simulink model "VINS"  (R2018a)
settings: Solver=FixedStepDiscrete  StartTime=0.0  StopTime=inf  FixedStep=1/Fs  RelTol=1e-3  EnableMultiTasking=on
PreLoadFcn:
  | modelDef = getModelDef(calibrateSFMA);
  | 
  | %imuPar = getImuPar('lmvpUncalibrated');
  | 
  | timeMatchThreshold = 1000;
undefined symbols (not defined in the file or in its folder): beep, dejitter_on, Fs, homogeneous3x4Transform_k_kmin1, imuLocationMm, imuPar, numStates, simData, tstamp_k_us, tstamp_kmin1_us
libraries: simulink x69, dspmtrx3 x35, dspindex x9, vrlib x7, dspstat3 x7, dspinverses x6, dspsigops x5, dspmathops x2, rtwdemowidgets x1, dspfactors x1, simulink_extras x1
(part 5 of 6)

== system VINS/measUpdate/absolutePoseUpdate/applyErrors/applyXstateErrors/reOrthonormalization ==
  note: from http://www.dtic.mil/dtic/tr/fulltext/u2/p003621.pdf page 12
  note: Cfixed = C + 0.5(I-CC')C
  In1 : Inport
  C*C' : Product  Multiplication=Matrix(*)
  C*C'1 : Product  Multiplication=Matrix(*)
  Constant : Constant  Value=eye(3)  OutDataTypeStr=Inherit: Inherit via back propagation
  Gain : Gain  Gain=1/2
  Permute Dimensions : PermuteDimensions
  Sum : Sum  Inputs=|++
  Sum1 : Sum  Inputs=|+-
  Out1 : Outport
  wires:
  In1/1 -> Permute Dimensions/1, C*C'/1, C*C'1/2, Sum/1
  Sum/1 -> Out1/1
  Permute Dimensions/1 -> C*C'/2
  C*C'/1 -> Sum1/2
  Constant/1 -> Sum1/1
  Gain/1 -> Sum/2
  Sum1/1 -> C*C'1/1
  C*C'1/1 -> Gain/1

== system VINS/measUpdate/absolutePoseUpdate/applyErrors/applyXstateErrors/updateAccelBiases ==
  In1 : Inport
  Enable : EnablePort
  Data Store Read5 : DataStoreRead  DataStoreName=df
  Data Store Write5 : DataStoreWrite  DataStoreName=df
  Sum4 : Sum  Inputs=++|
  wires:
  In1/1 -> Sum4/1
  Data Store Read5/1 -> Sum4/2
  Sum4/1 -> Data Store Write5/1

== system VINS/measUpdate/absolutePoseUpdate/applyErrors/applyXstateErrors/updateAccelSfma ==
  In1 : Inport
  Enable : EnablePort
  " LU Inverse" : dspinverses/ LU Inverse
      settings: SourceProductName=DSP System Toolbox
  Bias : Bias  Bias=eye(3)
  Data Store Read6 : DataStoreRead  DataStoreName=Macc
  Data Store Write6 : DataStoreWrite  DataStoreName=Macc
  Data Store Write9 : DataStoreWrite  DataStoreName=IplusMinv_acc
  Reshape : Reshape  OutputDimensionality=Customize  OutputDimensions=[3,3]
  Sum5 : Sum  Inputs=++|
  wires:
  " LU Inverse"/1 -> Data Store Write9/1
  Bias/1 -> " LU Inverse"/1
  In1/1 -> Reshape/1
  Reshape/1 -> Sum5/1
  Data Store Read6/1 -> Sum5/2
  Sum5/1 -> Data Store Write6/1, Bias/1

== system VINS/measUpdate/absolutePoseUpdate/applyErrors/applyXstateErrors/updateGyroGsensitivity ==
  In1 : Inport
  Enable : EnablePort
  Data Store Read7 : DataStoreRead  DataStoreName=Ggyr
  Data Store Write7 : DataStoreWrite  DataStoreName=Ggyr
  Reshape1 : Reshape  OutputDimensionality=Customize  OutputDimensions=[3,3]
  Sum6 : Sum  Inputs=++|
  wires:
  Data Store Read7/1 -> Sum6/2
  Reshape1/1 -> Sum6/1
  In1/1 -> Reshape1/1
  Sum6/1 -> Data Store Write7/1

== system VINS/measUpdate/absolutePoseUpdate/applyErrors/applyXstateErrors/updateGyroSfma ==
  In1 : Inport
  Enable : EnablePort
  " LU Inverse1" : dspinverses/ LU Inverse
      settings: SourceProductName=DSP System Toolbox
  Bias1 : Bias  Bias=eye(3)
  Data Store Read7 : DataStoreRead  DataStoreName=Mgyr
  Data Store Write7 : DataStoreWrite  DataStoreName=Mgyr
  Data Store Write8 : DataStoreWrite  DataStoreName=IplusMinv_gyr
  Reshape1 : Reshape  OutputDimensionality=Customize  OutputDimensions=[3,3]
  Sum6 : Sum  Inputs=++|
  wires:
  " LU Inverse1"/1 -> Data Store Write8/1
  Bias1/1 -> " LU Inverse1"/1
  Data Store Read7/1 -> Sum6/2
  Reshape1/1 -> Sum6/1
  In1/1 -> Reshape1/1
  Sum6/1 -> Data Store Write7/1, Bias1/1

== system VINS/measUpdate/relativePoseUpdate/applyErrors/applyErrors/For Each Subsystem ==
  delayedPoseCorrections : Inport  Partition=on  PartitionDimension=1  PartitionWidth=6  PartitionOffset=0
  C_c_n_list_in : Inport  Port=2  Partition=on  PartitionDimension=3  PartitionWidth=1  PartitionOffset=0
  r_c_n_list_in : Inport  Port=3  Partition=on  PartitionDimension=3  PartitionWidth=1  PartitionOffset=0
  Demux : Demux  Outputs=[3 3]
  For Each : ForEach  DisableCoverage=on  IndexMode=One-based
  Product2 : Product  Multiplication=Matrix(*)
  Sum : Sum  Inputs=++|
  Sum2 : Sum  Inputs=-+|
  reOrthonormalization : Subsystem  TreatAsAtomicUnit=on
  skew : MATLAB Function  TreatAsAtomicUnit=on
  C_c_n_list : Outport  ConcatenationDimension=3
  r_c_n_list : Outport  Port=2  ConcatenationDimension=3
  wires:
  delayedPoseCorrections/1 -> Demux/1
  Product2/1 -> Sum/1
  C_c_n_list_in/1 -> Sum/2, Product2/2
  reOrthonormalization/1(Out1) -> C_c_n_list/1
  skew/1(res) -> Product2/1  "[phi X]"
  Sum2/1 -> r_c_n_list/1
  r_c_n_list_in/1 -> Sum2/2
  Demux/1 -> skew/1(inp_vr)  "phi rotation errors"
  Demux/2 -> Sum2/1
  Sum/1 -> reOrthonormalization/1(In1)

== system VINS/measUpdate/relativePoseUpdate/applyErrors/applyErrors/applyXstateErrors ==
  errorStateEstimates : Inport
  Constant : Constant  Value=modelDef.trackGyroSfma
  Constant1 : Constant  Value=modelDef.trackAccelSfma
  Constant2 : Constant  Value=modelDef.trackAccelBiases
  Constant3 : Constant  Value=modelDef.trackGyroGsens
  Data Store Read1 : DataStoreRead  DataStoreName=dw
  Data Store Read2 : DataStoreRead  DataStoreName=Cbn
  Data Store Read3 : DataStoreRead  DataStoreName=rnav
  Data Store Read4 : DataStoreRead  DataStoreName=vnav
  Data Store Write1 : DataStoreWrite  DataStoreName=Cbn
  Data Store Write2 : DataStoreWrite  DataStoreName=dw
  Data Store Write3 : DataStoreWrite  DataStoreName=rnav
  Data Store Write4 : DataStoreWrite  DataStoreName=vnav
  Multiport Selector : dspindex/Multiport Selector  rowsOrCols=Rows  idxCellArray={ 1:3, 4:6, 7:9, 10:12, 13:15, 16:24, 25:33, 34:42 }  idxErrMode=Clip Index
  Product2 : Product  Multiplication=Matrix(*)
  Scope{,1..3} (4 alike) : Scope
  Sum : Sum  Inputs=++|
  Sum1 : Sum  Inputs=++|
  Sum2 : Sum  Inputs=-+|
  Sum3 : Sum  Inputs=-+|
  reOrthonormalization : Subsystem  TreatAsAtomicUnit=on
  skew : MATLAB Function  TreatAsAtomicUnit=on
  updateAccelBiases : Subsystem
  updateAccelSfma : Subsystem
  updateGyroGsensitivity : Subsystem
  updateGyroSfma : Subsystem
  wires:
  Multiport Selector/4 -> Sum3/1, Scope2/1
  Multiport Selector/3 -> Sum2/1, Scope1/1
  Sum3/1 -> Data Store Write4/1
  Data Store Read4/1 -> Sum3/2
  Data Store Read3/1 -> Sum2/2
  Sum2/1 -> Data Store Write3/1
  errorStateEstimates/1 -> Multiport Selector/1
  Multiport Selector/2 -> Sum1/1, Scope/1  "gyro bias errors"
  Sum1/1 -> Data Store Write2/1
  Data Store Read1/1 -> Sum1/2
  Multiport Selector/1 -> skew/1(inp_vr)  "phi rotation errors"
  reOrthonormalization/1(Out1) -> Data Store Write1/1
  Data Store Read2/1 -> Sum/2, Product2/2
  Sum/1 -> reOrthonormalization/1(In1)
  Product2/1 -> Sum/1
  skew/1(res) -> Product2/1  "[phi X]"
  Constant/1 -> updateGyroSfma/Enable
  Multiport Selector/6 -> updateGyroSfma/1(In1)
  Constant1/1 -> updateAccelSfma/Enable
  Multiport Selector/7 -> updateAccelSfma/1(In1)
  Multiport Selector/5 -> updateAccelBiases/1(In1), Scope3/1
  Constant2/1 -> updateAccelBiases/Enable
  Constant3/1 -> updateGyroGsensitivity/Enable
  Multiport Selector/8 -> updateGyroGsensitivity/1(In1)

== system VINS/measUpdate/relativePoseUpdate/get row indices/validateRecency/previousIndex ==
  idx2 : Inport
  Constant : Constant  Value=modelDef.maxNumDelayedPoses
  Constant1 : Constant  Value=uint8(1)
  Sum : Sum  Inputs=|-+
  Switch : Switch  Threshold=uint8(2)
  idx1 : Outport
  wires:
  idx2/1 -> Sum/2, Switch/2
  Constant/1 -> Switch/3
  Constant1/1 -> Sum/1
  Sum/1 -> Switch/1
  Switch/1 -> idx1/1  "idx1"

== system VINS/measUpdate/relativePoseUpdate/get row indices/validateRecency/previousIndex1 ==
  idx2 : Inport
  Constant : Constant  Value=modelDef.maxNumDelayedPoses
  Constant1 : Constant  Value=uint8(1)
  Sum : Sum  Inputs=|-+
  Switch : Switch  Threshold=uint8(2)
  idx1 : Outport
  wires:
  Switch/1 -> idx1/1  "idx1"
  Sum/1 -> Switch/1
  Constant1/1 -> Sum/1
  Constant/1 -> Switch/3
  idx2/1 -> Switch/2, Sum/2

== system VINS/measUpdate/relativePoseUpdate/updateCovariance/repairCovarianceAndWrite/lowerBoundDiagonal and reconstruct ==
  note: lower bound sigmas:
      |
      | phi:  1e-4 rad
      | dw:  20 deg/hr =1e-4 rad/s
      | dr: 1e-4 m
      | dv: 1e-4 m/s
      | df: max(imuPar.accelAlignUncert, imuPar.accelScaleUncert) * 9.8 m/s/s
  LDL' : Inport
  Create Diagonal Matrix : dspmtrx3/Create Diagonal Matrix
      settings: SourceProductName=DSP System Toolbox  SourceProductBaseCode=DS
  Extract Diagonal : dspmtrx3/Extract Diagonal
      settings: SourceProductName=DSP System Toolbox  SourceProductBaseCode=DS
  Extract Triangular Matrix : dspmtrx3/Extract Triangular Matrix  fcn=Lower  SimulateUsing=Code generation
      settings: SourceProductName=DSP System Toolbox  SourceProductBaseCode=DS
  Math Function : Math  Operator=square  SaturateOnIntegerOverflow=on
  Matrix Multiply : Product  Inputs=3  Multiplication=Matrix(*)
  Max : MinMax  Function=max  Inputs=2
  MinMax : MinMax
  MinMax1 : MinMax  Function=max
  Overwrite Values : dspmtrx3/Overwrite Values  OverWriteDiag=Diagonal  valFrom2ndIP=Second input port  ConstValue=0  RowSpan=Range of rows  RowStartMode=First  RowStartIndex=1  RowEndMode=Last  RowEndIndex=1  ColSpan=Range of columns  ColStartMode=First  ColStartIndex=1  ColEndMode=Last  ColEndIndex=1  DiagSpan=All elements  DiagStartMode=Index  DiagStartIndex=2  DiagEndMode=Index  DiagEndIndex=4
      settings: SourceProductName=DSP System Toolbox  SourceProductBaseCode=DS
  Permute Dimensions : PermuteDimensions
  Scope : Scope  NumInputPorts=2
  lowerBoundSigmas : Constant  Value="[1e-4 * ones(1,12)  9.8*max(imuPar.accelAlignUncert, imuPar.accelScaleUncert) * ones(1,3*modelDef.trackAccelBiases)   1e-4 * ones(1,modelDef.maxNumDelayedPoses*modelDef.statesPerDelayedPose)]"  OutDataTypeStr=Inherit: Inherit via back propagation
  ones size of diagonal : Product  Inputs=*/
  ones size of diagonal1 : Product  Inputs=*/
  rcond? : Scope
  P : Outport
  wires:
  Extract Diagonal/1 -> MinMax1/1, MinMax/1, Max/1, ones size of diagonal/2, ones size of diagonal/1
  Math Function/1 -> Max/2
  lowerBoundSigmas/1 -> Math Function/1
  LDL'/1 -> Extract Triangular Matrix/1, Extract Diagonal/1
  Extract Triangular Matrix/1 -> Overwrite Values/1
  ones size of diagonal/1 -> Overwrite Values/2
  Overwrite Values/1 -> Permute Dimensions/1, Matrix Multiply/1  "L"
  Matrix Multiply/1 -> P/1
  Permute Dimensions/1 -> Matrix Multiply/3  "L'"
  Create Diagonal Matrix/1 -> Matrix Multiply/2
  MinMax/1 -> ones size of diagonal1/1, Scope/1
  MinMax1/1 -> ones size of diagonal1/2, Scope/2
  ones size of diagonal1/1 -> rcond?/1
  Max/1 -> Create Diagonal Matrix/1

== system VINS/measUpdate/relativePoseUpdate/updateCovariance/writeCovariances/lowerBoundStates ==
  note: lower bound sigmas:
      |
      | phi:  1e-4 rad
      | dw:  20 deg/hr =1e-4 rad/s
      | dr: 1e-4 m
      | dv: 1e-4 m/s
      | df: max(imuPar.accelAlignUncert, imuPar.accelScaleUncert) * 9.8 m/s/s
  In1 : Inport
  Extract Diagonal : dspmtrx3/Extract Diagonal
      settings: SourceProductName=DSP System Toolbox  SourceProductBaseCode=DS
  Math Function : Math  Operator=square  SaturateOnIntegerOverflow=on
  Max : MinMax  Function=max  Inputs=2
  Overwrite Values : dspmtrx3/Overwrite Values  OverWriteDiag=Diagonal  valFrom2ndIP=Second input port  ConstValue=0  RowSpan=Range of rows  RowStartMode=First  RowStartIndex=1  RowEndMode=Last  RowEndIndex=1  ColSpan=Range of columns  ColStartMode=First  ColStartIndex=1  ColEndMode=Last  ColEndIndex=1  DiagSpan=All elements  DiagStartMode=Index  DiagStartIndex=2  DiagEndMode=Index  DiagEndIndex=4
      settings: SourceProductName=DSP System Toolbox  SourceProductBaseCode=DS
  lowerBoundSigmas : Constant  Value="[1e-4 * ones(1,12)  9.8*max(imuPar.accelAlignUncert, imuPar.accelScaleUncert) * ones(1,3)]"  OutDataTypeStr=Inherit: Inherit via back propagation
  Out1 : Outport
  wires:
  In1/1 -> Overwrite Values/1, Extract Diagonal/1
  lowerBoundSigmas/1 -> Math Function/1
  Extract Diagonal/1 -> Max/1
  Math Function/1 -> Max/2
  Max/1 -> Overwrite Values/2
  Overwrite Values/1 -> Out1/1

== system VINS/measUpdate/relativePoseUpdate/updateCovariance/writeCovariances/lowerBoundStates1 ==
  note: lower bound sigmas:
      |
      | phi:  1e-4 rad
      | dw:  20 deg/hr =1e-4 rad/s
      | dr: 1e-4 m
      | dv: 1e-4 m/s
      | df: max(imuPar.accelAlignUncert, imuPar.accelScaleUncert) * 9.8 m/s/s
  In1 : Inport
  Extract Diagonal : dspmtrx3/Extract Diagonal
      settings: SourceProductName=DSP System Toolbox  SourceProductBaseCode=DS
  Math Function : Math  Operator=square  SaturateOnIntegerOverflow=on
  Max : MinMax  Function=max  Inputs=2
  Overwrite Values : dspmtrx3/Overwrite Values  OverWriteDiag=Diagonal  valFrom2ndIP=Second input port  ConstValue=0  RowSpan=Range of rows  RowStartMode=First  RowStartIndex=1  RowEndMode=Last  RowEndIndex=1  ColSpan=Range of columns  ColStartMode=First  ColStartIndex=1  ColEndMode=Last  ColEndIndex=1  DiagSpan=All elements  DiagStartMode=Index  DiagStartIndex=2  DiagEndMode=Index  DiagEndIndex=4
      settings: SourceProductName=DSP System Toolbox  SourceProductBaseCode=DS
  lowerBoundSigmas : Constant  Value="[  1e-4 * ones(1,modelDef.maxNumDelayedPoses*modelDef.statesPerDelayedPose) ]"  OutDataTypeStr=Inherit: Inherit via back propagation
  Out1 : Outport
  wires:
  Overwrite Values/1 -> Out1/1
  Max/1 -> Overwrite Values/2
  Math Function/1 -> Max/2
  Extract Diagonal/1 -> Max/1
  lowerBoundSigmas/1 -> Math Function/1
  In1/1 -> Extract Diagonal/1, Overwrite Values/1

== system VINS/measUpdate/relocalize/Subsystem/setPosition/DT police3 ==
  In1 : Inport
  Data Store Read : DataStoreRead  DataStoreName=DataTypeRef
  Data Type Duplicate : DataTypeDuplicate
  wires:
  Data Store Read/1 -> Data Type Duplicate/1
  In1/1 -> Data Type Duplicate/2

== system VINS/measUpdate/relativePoseUpdate/applyErrors/applyErrors/For Each Subsystem/reOrthonormalization ==
  note: Cfixed = C + 0.5(I-CC')C
  note: from http://www.dtic.mil/dtic/tr/fulltext/u2/p003621.pdf page 12
  In1 : Inport
  C*C' : Product  Multiplication=Matrix(*)
  C*C'1 : Product  Multiplication=Matrix(*)
  Constant : Constant  Value=eye(3)  OutDataTypeStr=Inherit: Inherit via back propagation
  Gain : Gain  Gain=1/2
  Permute Dimensions : PermuteDimensions
  Sum : Sum  Inputs=|++
  Sum1 : Sum  Inputs=|+-
  Out1 : Outport
  wires:
  C*C'1/1 -> Gain/1
  Sum1/1 -> C*C'1/1
  Gain/1 -> Sum/2
  Constant/1 -> Sum1/1
  C*C'/1 -> Sum1/2
  Permute Dimensions/1 -> C*C'/2
  Sum/1 -> Out1/1
  In1/1 -> Sum/1, C*C'1/2, C*C'/1, Permute Dimensions/1

== system VINS/measUpdate/relativePoseUpdate/applyErrors/applyErrors/applyXstateErrors/reOrthonormalization ==
  note: Cfixed = C + 0.5(I-CC')C
  note: from http://www.dtic.mil/dtic/tr/fulltext/u2/p003621.pdf page 12
  In1 : Inport
  C*C' : Product  Multiplication=Matrix(*)
  C*C'1 : Product  Multiplication=Matrix(*)
  Constant : Constant  Value=eye(3)  OutDataTypeStr=Inherit: Inherit via back propagation
  Gain : Gain  Gain=1/2
  Permute Dimensions : PermuteDimensions
  Sum : Sum  Inputs=|++
  Sum1 : Sum  Inputs=|+-
  Out1 : Outport
  wires:
  C*C'1/1 -> Gain/1
  Sum1/1 -> C*C'1/1
  Gain/1 -> Sum/2
  Constant/1 -> Sum1/1
  C*C'/1 -> Sum1/2
  Permute Dimensions/1 -> C*C'/2
  Sum/1 -> Out1/1
  In1/1 -> Sum/1, C*C'1/2, C*C'/1, Permute Dimensions/1

== system VINS/measUpdate/relativePoseUpdate/applyErrors/applyErrors/applyXstateErrors/updateAccelBiases ==
  In1 : Inport
  Enable : EnablePort
  Data Store Read5 : DataStoreRead  DataStoreName=df
  Data Store Write5 : DataStoreWrite  DataStoreName=df
  Sum4 : Sum  Inputs=++|
  wires:
  Sum4/1 -> Data Store Write5/1
  Data Store Read5/1 -> Sum4/2
  In1/1 -> Sum4/1

== system VINS/measUpdate/relativePoseUpdate/applyErrors/applyErrors/applyXstateErrors/updateAccelSfma ==
  In1 : Inport
  Enable : EnablePort
  " LU Inverse" : dspinverses/ LU Inverse
      settings: SourceProductName=DSP System Toolbox
  Bias : Bias  Bias=eye(3)
  Data Store Read6 : DataStoreRead  DataStoreName=Macc
  Data Store Write6 : DataStoreWrite  DataStoreName=Macc
  Data Store Write9 : DataStoreWrite  DataStoreName=IplusMinv_acc
  Reshape : Reshape  OutputDimensionality=Customize  OutputDimensions=[3,3]
  Sum5 : Sum  Inputs=++|
  wires:
  Sum5/1 -> Bias/1, Data Store Write6/1
  Data Store Read6/1 -> Sum5/2
  Reshape/1 -> Sum5/1
  In1/1 -> Reshape/1
  Bias/1 -> " LU Inverse"/1
  " LU Inverse"/1 -> Data Store Write9/1

== system VINS/measUpdate/relativePoseUpdate/applyErrors/applyErrors/applyXstateErrors/updateGyroGsensitivity ==
  In1 : Inport
  Enable : EnablePort
  Data Store Read7 : DataStoreRead  DataStoreName=Ggyr
  Data Store Write7 : DataStoreWrite  DataStoreName=Ggyr
  Reshape1 : Reshape  OutputDimensionality=Customize  OutputDimensions=[3,3]
  Sum6 : Sum  Inputs=++|
  wires:
  Sum6/1 -> Data Store Write7/1
  In1/1 -> Reshape1/1
  Reshape1/1 -> Sum6/1
  Data Store Read7/1 -> Sum6/2

== system VINS/measUpdate/relativePoseUpdate/applyErrors/applyErrors/applyXstateErrors/updateGyroSfma ==
  In1 : Inport
  Enable : EnablePort
  " LU Inverse1" : dspinverses/ LU Inverse
      settings: SourceProductName=DSP System Toolbox
  Bias1 : Bias  Bias=eye(3)
  Data Store Read7 : DataStoreRead  DataStoreName=Mgyr
  Data Store Write7 : DataStoreWrite  DataStoreName=Mgyr
  Data Store Write8 : DataStoreWrite  DataStoreName=IplusMinv_gyr
  Reshape1 : Reshape  OutputDimensionality=Customize  OutputDimensions=[3,3]
  Sum6 : Sum  Inputs=++|
  wires:
  Sum6/1 -> Bias1/1, Data Store Write7/1
  In1/1 -> Reshape1/1
  Reshape1/1 -> Sum6/1
  Data Store Read7/1 -> Sum6/2
  Bias1/1 -> " LU Inverse1"/1
  " LU Inverse1"/1 -> Data Store Write8/1

== matlab function VINS/stilltimes/updateStilltimeTight ==
  data: w input; stilltime output; f input; Dt input; favgs output; wavgs output; wsigma input; fsigma input
function [stilltime, favgs, wavgs] = update_stilltime(w, f, Dt, wsigma, fsigma)

persistent stillt wavg favg stillcycles wsigmas fsigmas;

if isempty(wavg)
    stillt = cast(0, 'like', w);
    stillcycles = cast(0, 'like', w);
    wavg = w;
    favg = f;
    wsigmas = wsigma*cast([1;1;1], 'like', w);
    fsigmas = fsigma*cast([1;1;1], 'like', w);
end

if all(abs(f-favg) < 3*fsigmas) && all(abs(w-wavg) < 3*wsigmas)  % increment the stilltimes
    stillt = stillt + Dt;
    stillcycles = stillcycles + cast(1, 'like', w);
%     % simple recursive mean (weighting all the samples equally):
%     wavg = ((stillcycles-1)*wavg + w)/stillcycles;
%     favg = ((stillcycles-1)*favg + f)/stillcycles;

%     % recursive mean with each sample weighted by the stillcycles when it came in:
%     wavg = ((stillcycles-1)*wavg + 2*w)/(stillcycles+1);
%     favg = ((stillcycles-1)*favg + 2*f)/(stillcycles+1);

    % start with stillcycles weighting and switch back to simple recursive mean after 1 second to reduce noise:
    if stillt < 1
        wavg = ((stillcycles-cast(1, 'like', w))*wavg + 2*w)/(stillcycles+cast(1, 'like', w));
        favg = ((stillcycles-1)*favg + 2*f)/(stillcycles+1);
    else
        wavg = ((stillcycles-1)*wavg + w)/stillcycles;
        favg = ((stillcycles-1)*favg + f)/stillcycles;
    end        
else  %reset stilltime
    stillt = cast(0, 'like', w);
    stillcycles = cast(0, 'like', w);
    wavg = w;
    favg = f;
end    

stilltime = stillt;
favgs = favg;
wavgs = wavg;

== matlab function VINS/reportOutputs/MATLAB Function3 ==
  data: Cbn input; eul output size=[3,1]
function eul = dcm2euler(Cbn)

%DCM is Cbn (transforms vectors from b to n)
%eul defined as zyx sequence (yaw,pitch,roll),  but listed in
%roll,pitch,yaw order


pitch=asin(-Cbn(3,1));  %pitch is assumed to be [-pi pi]. singular at pi. use ad-hoc methods to remedy this deficiency
roll=atan2(Cbn(3,2), Cbn(3,3));
heading = atan2(Cbn(2,1), Cbn(1,1));
eul=[roll;pitch;heading];

== matlab function VINS/measUpdate/gravity meas update/update the Cbn and b_g with the errors/MATLAB Function ==
  data: inp_vr input; res output
function res=skew(inp_vr)
res=[0 			-inp_vr(3)	inp_vr(2); ...
     inp_vr(3)	0			-inp_vr(1);...
	 -inp_vr(2)	inp_vr(1)	0];

== matlab function VINS/measUpdate/gravity meas update/MATLAB Function1 ==
  data: S output; P input; K output; H input; R input
function [S,K] = calcKalmanGain(P, H, R)

PHT = P*H';
S = H*PHT + R;
K = PHT/S;

== matlab function VINS/uncomment and set zero noise for verification/plot errors/MATLAB Function3 ==
  data: Cbn input; eul output size=[3,1]
function eul = dcm2euler(Cbn)

%DCM is Cbn (transforms vectors from b to n)
%eul defined as zyx sequence (yaw,pitch,roll),  but listed in
%roll,pitch,yaw order


pitch=asin(-Cbn(3,1));  %pitch is assumed to be [-pi pi]. singular at pi. use ad-hoc methods to remedy this deficiency
roll=atan2(Cbn(3,2), Cbn(3,3));
heading = atan2(Cbn(2,1), Cbn(1,1));
eul=[roll;pitch;heading];

== matlab function VINS/timeUpdate/calculateQ ==
  data: omega input; Q output size=[modelDef.numStates, modelDef.numStates]; f_ib input; Dt input; Cbn input; modelDef parameter; imuPar parameter
function Q  = calculate_Q(omega, f_ib, Dt, Cbn, modelDef, imuPar)

% order of the states:
% 1:3   phi
% 4:6   dw
% 7:9   dr
% 10:12 dv
% 13:15 df  (if modelDef.trackAccelBiases)
% 16:24 dM_gyro in column-major order (if modelDef.trackGyroSfma)
% 25:33 dM_accel in column-major order (if modelDef.trackAccelSfma)

Q = zeros(modelDef.numStates, 'like', omega);

omega = reshape(omega,3,1); 
f_ib = reshape(f_ib, 3,1);

Qphi = diag((imuPar.gyroArwRadPerRtSec^2)*[Dt Dt Dt]);  
Qdw = diag((imuPar.gyroBrwRadPerSecPerRtSec^2)*[Dt Dt Dt]);
Qdv = diag((imuPar.accelVrwMetersPerSecPerRtSec^2)*[Dt Dt Dt]);
Qdf = diag((imuPar.accelBrwMetersPerSec2PerRtSec^2)*[Dt Dt Dt]);


%bump up Q for unmodelled states
if ~modelDef.trackGyroSfma % gyro scale factor and misalignment not tracked
   gyroSfSigmaBod = imuPar.gyroScaleUncert*omega;
   gyroMaSigmaBod = imuPar.gyroAlignUncert*sqrt(omega'*omega*[1 1 1]-omega'.*omega');   
   QgyroMa = Cbn*diag(gyroMaSigmaBod.^2)*Cbn'*Dt; 
   QgyroSf = Cbn*diag(gyroSfSigmaBod.^2)*Cbn'*Dt; 
   Qphi = Qphi + QgyroMa + QgyroSf;   
end

if ~modelDef.trackGyroGsens %  gyro g sensitivity not tracked 
   gGsensSigmaBod = imuPar.gyroGsensUncert*sqrt(f_ib'*f_ib*[1 1 1]-f_ib'.*f_ib');   
   QgGsens = Cbn*diag(gGsensSigmaBod.^2)*Cbn'*Dt; 
   Qphi = Qphi + QgGsens;   
end

if ~modelDef.trackAccelSfma  % accel scale factor and misalignment not tracked
    %original form
   accelSfSigmaBod = imuPar.accelScaleUncert*f_ib;
   accelMaSigmaBod = imuPar.accelAlignUncert*sqrt(f_ib'*f_ib*[1 1 1]-f_ib'.*f_ib');   
   QaccelMa = Cbn*diag(accelMaSigmaBod.^2)*Cbn'*Dt; 
   QaccelSf = Cbn*diag(accelSfSigmaBod.^2)*Cbn'*Dt; 
   Qdv = Qdv + 50*(QaccelMa + QaccelSf);     
%new form (doesn't work):
%    ffT = f_ib * f_ib';
%    accelSfSigma = imuPar.accelScaleUncert;
%    accelMaSigma = imuPar.accelAlignUncert;
%    fmagn2 = f_ib'*f_ib;
%    QaccelMa = Cbn*(accelMaSigma^2 * (ffT + fmagn2*eye(3) - 2*diag(f_ib.*f_ib)))*Cbn'*Dt; 
%    QaccelSf = Cbn*(accelSfSigma^2 * ffT)*Cbn'*Dt; 
%    Qdv = Qdv + QaccelMa + QaccelSf;  
 % simpler form:
%     fmagn2 = f_ib'*f_ib;
%     Qdv = Qdv + 100*Dt * eye(3) * fmagn2 * max(imuPar.accelScaleUncert, imuPar.accelAlignUncert)^2;

end

if ~modelDef.trackAccelBiases
   accelBiasSigmaBod = imuPar.accelBiasUncert*[1;1;1];
   QaccelBias = Cbn*diag(accelBiasSigmaBod.^2)*Cbn'*Dt; 
   Qdv = Qdv + 100*(QaccelBias);     
end

Q(1:3, 1:3) = Qphi;
Q(4:6, 4:6) = Qdw;
Q(10:12, 10:12) = Qdv;
if modelDef.trackAccelBiases
    Q(13:15, 13:15) = Qdf;
end

== matlab function VINS/timeUpdate/MATLAB Function1 ==
  data: imuPar output Bus: imuPar
function imuPar = imuPar

imuPar.gyroArwDegPerRtHr = 0.25;
imuPar.gyroArwRadPerRtSec = imuPar.gyroArwDegPerRtHr * pi/180/60;
imuPar.gyroBrwDegPerHrPerRtHr = 0;
imuPar.gyroBrwRadPerSecPerRtSec = imuPar.gyroBrwDegPerHrPerRtHr * pi/180/3600/60;
imuPar.gyroScaleUncertainty = 0.001;
imuPar.gyroAlignUncertainty = 0.01;
imuPar.gyroGsensUncertainty = 0.001;

== matlab function VINS/timeUpdate/MATLAB Function2 ==
  settings: updateMethod=DISCRETE  sampleTime=inf
  data: modelDef output Bus: modelDef; numStates input
function modelDef = modelDef(numStates)

modelDef.trackAccelBiases = true;
modelDef.trackAccelSfma = true;
modelDef.trackGyroSfma = true;
modelDef.trackGyroGsens = false;

modelDef.numStates = numStates;

== matlab function VINS/timeUpdate/calculatePhi ==
  data: omega input; Phi output size=[modelDef.numStates, modelDef.numStates]; fbod input; Dt input; Cbn input; modelDef parameter
function Phi  = calculate_Phi(omega, fbod, Dt, Cbn, modelDef)

% order of the states:
% 1:3   phi
% 4:6   dw
% 7:9   dr
% 10:12 dv
% 13:15 df  (if modelDef.trackAccelBiases)
% 16:24 dM_gyro in column-major order (if modelDef.trackGyroSfma)
% 25:33 dM_accel in column-major order (if modelDef.trackAccelSfma)
% 34:42 dG_gyro in column-major order (if modelDef.trackGyroGsens)

Phi = eye(modelDef.numStates, 'like', omega);

DtC = Dt*Cbn;

Phi(1:3,4:6) = -DtC;  % propagate dw to phi
Phi(7:9, 10:12) = Dt*eye(3, 'like', omega);  % propagate dv to dr
Phi(10:12, 1:3) = Dt*skew(Cbn*fbod);  % propagate phi to dv

if modelDef.trackAccelBiases
    Phi(10:12, 13:15) = DtC;   % propagate df to dv
end

if modelDef.trackGyroSfma  % propagate dM_gyro to phi
    Phi(1:3, 16:18) = -DtC*omega(1);
    Phi(1:3, 19:21) = -DtC*omega(2);
    Phi(1:3, 22:24) = -DtC*omega(3);
end

if modelDef.trackAccelSfma  % propagate dM_accel to dv
    Phi(10:12, 25:27) = DtC*fbod(1);
    Phi(10:12, 28:30) = DtC*fbod(2);
    Phi(10:12, 31:33) = DtC*fbod(3);
end

if modelDef.trackGyroGsens  % propagate dG_gyro to phi
    Phi(1:3, 34:36) = -DtC*fbod(1);
    Phi(1:3, 37:39) = -DtC*fbod(2);
    Phi(1:3, 40:42) = -DtC*fbod(3);
end


function res=skew(inp_vr)
res=[0 			-inp_vr(3)	inp_vr(2); ...
     inp_vr(3)	0			-inp_vr(1);...
	 -inp_vr(2)	inp_vr(1)	0];

== matlab function VINS/measUpdate/zuptMeasUpdate/calculateKalmanGain ==
  data: S output; P input; K output; H input; R input
function [S,K] = calcKalmanGain(P, H, R)

PHT = P*H';
S = H*PHT + R;
K = PHT/S;

== matlab function VINS/stilltimes/updateStilltimeLoose ==
  data: w input; stilltime output; f input; Dt input; favgs output; wavgs output; wsigma input; fsigma input
function [stilltime, favgs, wavgs] = update_stilltime(w, f, Dt, wsigma, fsigma)

persistent stillt wavg favg stillcycles wsigmas fsigmas;

if isempty(wavg)
    stillt = cast(0, 'like', w);
    stillcycles = cast(0, 'like', w);
    wavg = w;
    favg = f;
    wsigmas = wsigma*cast([1;1;1], 'like', w);
    fsigmas = fsigma*cast([1;1;1], 'like', w);
end

if all(abs(f-favg) < 3*fsigmas) && all(abs(w-wavg) < 3*wsigmas)  % increment the stilltimes
    stillt = stillt + Dt;
    stillcycles = stillcycles + cast(1, 'like', w);
%     % simple recursive mean (weighting all the samples equally):
%     wavg = ((stillcycles-1)*wavg + w)/stillcycles;
%     favg = ((stillcycles-1)*favg + f)/stillcycles;

%     % recursive mean with each sample weighted by the stillcycles when it came in:
%     wavg = ((stillcycles-1)*wavg + 2*w)/(stillcycles+1);
%     favg = ((stillcycles-1)*favg + 2*f)/(stillcycles+1);

    % start with stillcycles weighting and switch back to simple recursive mean after 1 second to reduce noise:
    if stillt < 1
        wavg = ((stillcycles-cast(1, 'like', w))*wavg + 2*w)/(stillcycles+cast(1, 'like', w));
        favg = ((stillcycles-1)*favg + 2*f)/(stillcycles+1);
    else
        wavg = ((stillcycles-1)*wavg + w)/stillcycles;
        favg = ((stillcycles-1)*favg + f)/stillcycles;
    end        
else  %reset stilltime
    stillt = cast(0, 'like', w);
    stillcycles = cast(0, 'like', w);
    wavg = w;
    favg = f;
end    

stilltime = stillt;
favgs = favg;
wavgs = wavg;

== matlab function VINS/initStatesCovariances/setP/MATLAB Function1 ==
  data: initialRotUncert input; initialPosUncert input; initialVelUncert input; P0 output size=[modelDef.numStates, modelDef.numStates]; modelDef parameter; imuPar parameter
function P0  = calculate_P0(initialRotUncert, initialPosUncert, initialVelUncert, modelDef, imuPar)

% order of the states:
% 1:3   phi
% 4:6   dw
% 7:9   dr
% 10:12 dv
% 13:15 df  (if modelDef.trackAccelBiases)
% 16:24 dM_gyro in column-major order (if modelDef.trackGyroSfma)
% 25:33 dM_accel in column-major order (if modelDef.trackAccelSfma)
% 34:42 dG_gyro in column-major order (if modelDef.trackGyroGsens)

P0 = zeros(modelDef.numStates, 'like', initialRotUncert);

P0(1:3, 1:3) = diag(initialRotUncert.^2);
P0(4:6, 4:6) = eye(3)*(imuPar.gyroBiasUncert.^2);
P0(7:9, 7:9) = diag(initialPosUncert.^2);
P0(10:12, 10:12) = diag(initialVelUncert.^2);


if modelDef.trackAccelBiases
    P0(13:15, 13:15) = eye(3)*(imuPar.accelBiasUncert.^2);
end

if modelDef.trackGyroSfma  
    vec9 = ones(9,1)*imuPar.gyroAlignUncert^2;
    vec9([1 5 9]) = imuPar.gyroScaleUncert^2;
    P0(16:24, 16:24) = diag(vec9);
end

if modelDef.trackAccelSfma  % propagate dM_accel to dv
    vec9 = ones(9,1)*imuPar.accelAlignUncert^2;
    vec9([1 5 9]) = imuPar.accelScaleUncert^2;
    if modelDef.accelDefinesExtrinsics
        vec9([4 7]) = 0.0001^2; % x accel has no misalignment so picks up no component of y or z accelerations
        vec9(8) = 0.0001^2;  % y accel has no tilt out of xy plane, so picks up no component of z acceleration
    end
    P0(25:33, 25:33) = diag(vec9);
end

if modelDef.trackGyroGsens
    vec9 = ones(9,1)*imuPar.gyroGsensUncert^2;
    P0(34:42, 34:42) = diag(vec9);
end

== matlab function VINS/measUpdate/gravity meas update/MATLAB Function3 ==
  data: P input; Pplus output; K input; H input; R input; IminKH output
function [Pplus, IminKH] = josephCovarianceUpdate(P, K, H, R)

IminKH = eye(size(P)) - K*H;
Pplus = IminKH*P*IminKH' + K*R*K';

== matlab function VINS/measUpdate/zuptMeasUpdate/josephCovarianceUpdate ==
  data: P input; Pplus output; K input; H input; R input; IminKH output
function [Pplus, IminKH] = josephCovarianceUpdate(P, K, H, R)

IminKH = eye(size(P), 'like', P) - K*H;
Pplus = IminKH*P*IminKH' + K*R*K';

== matlab function VINS/measUpdate/zuptMeasUpdate/applyErrors/skew ==
  data: inp_vr input; res output
function res=skew(inp_vr)
res=[cast(0, 'like', inp_vr)	-inp_vr(3)                  inp_vr(2); ...
     inp_vr(3)                  cast(0, 'like', inp_vr)     -inp_vr(1);...
	 -inp_vr(2)                 inp_vr(1)                   cast(0, 'like', inp_vr)];

== matlab function VINS/reportOutputs/MATLAB Function1 ==
  data: Cbn input; quat output size=[4,1]
function quat=dcm2quat(Cbn)

%dcm (Cba) to quaternion (qba)
%Cba:B to A transformation matrix
%qba:B to A quaternion

%Implementation of savage(3-47)


tr=Cbn(1,1)+Cbn(2,2)+Cbn(3,3);
Pa=1+tr;
Pb=1+2*Cbn(1,1)-tr;
Pc=1+2*Cbn(2,2)-tr;
Pd=1+2*Cbn(3,3)-tr;

quat=zeros(4,1);
if (Pa>=Pb && Pa>=Pc && Pa>=Pd)
    quat(1)=0.5*sqrt(Pa);
    quat(2)=(Cbn(3,2)-Cbn(2,3))/4/quat(1);
    quat(3)=(Cbn(1,3)-Cbn(3,1))/4/quat(1);
    quat(4)=(Cbn(2,1)-Cbn(1,2))/4/quat(1);
elseif (Pb>=Pc && Pb>=Pd)
    quat(2)=0.5*sqrt(Pb);
    quat(3)=(Cbn(2,1)+Cbn(1,2))/4/quat(2);
    quat(4)=(Cbn(1,3)+Cbn(3,1))/4/quat(2);
    quat(1)=(Cbn(3,2)-Cbn(2,3))/4/quat(2);
elseif (Pc>=Pd)
    quat(3)=0.5*sqrt(Pc);
    quat(4)=(Cbn(3,2)+Cbn(2,3))/4/quat(3);
    quat(1)=(Cbn(1,3)-Cbn(3,1))/4/quat(3);
    quat(2)=(Cbn(2,1)+Cbn(1,2))/4/quat(3);
else
    quat(4)=0.5*sqrt(Pd);
    quat(1)=(Cbn(2,1)-Cbn(1,2))/4/quat(4);
    quat(2)=(Cbn(1,3)+Cbn(3,1))/4/quat(4);
    quat(3)=(Cbn(3,2)+Cbn(2,3))/4/quat(4);
end

if (quat(1)<=0)
    quat=-quat;
end

== matlab function VINS/augmentState/covarianceAugmentation ==
  data: indexToReplace input; Pxx input; Pxc input; Pcc input; r_bc_n input; Pxc output; Pcc output
function [Pxc, Pcc] = covarianceAugmentation(indexToReplace, Pxx, Pxc, Pcc, r_bc_n)


% Jx = [eye(3)     zeros(3) zeros(3) zeros(3) zeros(3); ...
%       zeros(3)   zeros(3) eye(3)   zeros(3) zeros(3)]

% calculate Pxx * Jx'
Pcol1  = Pxx(:,1:3);
Pcol3  = Pxx(:,7:9);
S = skew(r_bc_n);
PxxJxT = [Pcol1  Pcol3];

% calculate Jx * Pxx * Jx'
P11 = Pxx(1:3,1:3);
P13 = Pxx(1:3,7:9);
P33 = Pxx(7:9,7:9);

JxPxxJxT = [P11  P13; P13'  P33];

% calculate Jx * Pxc
JxPxc = [ Pxc(1:3,:) ; Pxc(7:9,:) ];

% now insert the new camera pose covariances into the rows of the pose to
% be replaced:
replaceIdx = uint8(6)*(indexToReplace-uint8(1)) + uint8(1:6);

Pxc(:,replaceIdx) = PxxJxT;
Pcc(replaceIdx,:) = JxPxc;
Pcc(:,replaceIdx) = JxPxc';
Pcc(replaceIdx,replaceIdx) = JxPxxJxT;
end

function res=skew(inp_vr)
res=[cast(0, 'like', inp_vr)	-inp_vr(3)                  inp_vr(2); ...
     inp_vr(3)                  cast(0, 'like', inp_vr)     -inp_vr(1);...
	 -inp_vr(2)                 inp_vr(1)                   cast(0, 'like', inp_vr)];
end

== matlab function VINS/measUpdate/relativePoseUpdate/applyErrors/applyErrors/applyXstateErrors/skew ==
  data: inp_vr input; res output
function res=skew(inp_vr)
res=[cast(0, 'like', inp_vr)	-inp_vr(3)                  inp_vr(2); ...
     inp_vr(3)                  cast(0, 'like', inp_vr)     -inp_vr(1);...
	 -inp_vr(2)                 inp_vr(1)                   cast(0, 'like', inp_vr)];

== matlab function VINS/measUpdate/relativePoseUpdate/calculateKalmanGain ==
  data: chiSquared output; P input; K output; H input; R input; RbumpedUp input; nu input
function [chiSquared,K] = calcKalmanGain(P, H, R, RbumpedUp, nu)

PHT = P*H';
HPHT = H*PHT;

S = HPHT + RbumpedUp;  % bump up the R to account for unmodelled colored noise sources due to camera calibration etc.
K = PHT/S;

S = HPHT + R;  % use a non-inflated meas noise for gating the measurements
chiSquared = nu' * (S \ nu);

== matlab function VINS/measUpdate/relativePoseUpdate/updateCovariance/josephCovarianceUpdate ==
  data: P input; Pplus output; K input; H input; R input; IminKH output
function [Pplus, IminKH] = josephCovarianceUpdate(P, K, H, R)

IminKH = eye(size(P), 'like', P) - K*H;
Pplus = IminKH*P*IminKH' + K*R*K';


% re-symmetrize:
Pplus = (Pplus + Pplus')/2;
% Pdiag = max(0.001^2, diag(Pplus));
% nrows = size(Pplus,1);
% 
% Pplus(1:(nrows+1):end) = Pdiag;  %this overwrites only the diagonal elements

== matlab function VINS/measUpdate/relativePoseUpdate/formInnovation/MATLAB Function3 ==
  data: Cbn input; eul output size=[3,1]
function eul = dcm2euler(Cbn)

%DCM is Cbn (transforms vectors from b to n)
%eul defined as zyx sequence (yaw,pitch,roll),  but listed in
%roll,pitch,yaw order


pitch=asin(-Cbn(3,1));  %pitch is assumed to be [-pi pi]. singular at pi. use ad-hoc methods to remedy this deficiency
roll=atan2(Cbn(3,2), Cbn(3,3));
heading = atan2(Cbn(2,1), Cbn(1,1));
eul=[roll;pitch;heading];

== matlab function VINS/measUpdate/relativePoseUpdate/applyErrors/applyErrors/For Each Subsystem/skew ==
  data: inp_vr input; res output
function res=skew(inp_vr)
res=[cast(0, 'like', inp_vr)	-inp_vr(3)                  inp_vr(2); ...
     inp_vr(3)                  cast(0, 'like', inp_vr)     -inp_vr(1);...
	 -inp_vr(2)                 inp_vr(1)                   cast(0, 'like', inp_vr)];

== matlab function VINS/measUpdate/relativePoseUpdate/formMeasurementMatrix/skew ==
  data: inp_vr input; res output
function res=skew(inp_vr)
res=[cast(0, 'like', inp_vr)	-inp_vr(3)                  inp_vr(2); ...
     inp_vr(3)                  cast(0, 'like', inp_vr)     -inp_vr(1);...
	 -inp_vr(2)                 inp_vr(1)                   cast(0, 'like', inp_vr)];

== matlab function VINS/initStatesCovariances/realInit/calcCbn/MATLAB Function3 ==
  data: Cbn input; eul output size=[3,1]
function eul = dcm2euler(Cbn)

%DCM is Cbn (transforms vectors from b to n)
%eul defined as zyx sequence (yaw,pitch,roll),  but listed in
%roll,pitch,yaw order


pitch=asin(-Cbn(3,1));  %pitch is assumed to be [-pi pi]. singular at pi. use ad-hoc methods to remedy this deficiency
roll=atan2(Cbn(3,2), Cbn(3,3));
heading = atan2(Cbn(2,1), Cbn(1,1));
eul=[roll;pitch;heading];

== matlab function VINS/measUpdate/absolutePoseUpdate/applyErrors/For Each Subsystem/skew ==
  data: inp_vr input; res output
function res=skew(inp_vr)
res=[cast(0, 'like', inp_vr)	-inp_vr(3)                  inp_vr(2); ...
     inp_vr(3)                  cast(0, 'like', inp_vr)     -inp_vr(1);...
	 -inp_vr(2)                 inp_vr(1)                   cast(0, 'like', inp_vr)];

== matlab function VINS/measUpdate/gravity meas update/MATLAB Function2 ==
  data: inp_vr input; res output
function res=skew(inp_vr)
res=[0 			-inp_vr(3)	inp_vr(2); ...
     inp_vr(3)	0			-inp_vr(1);...
	 -inp_vr(2)	inp_vr(1)	0];

== matlab function VINS/measUpdate/compass meas update/MATLAB Function1 ==
  data: S output; P input; K output; H input; R input
function [S,K] = calcKalmanGain(P, H, R)

PHT = P*H';
S = H*PHT + R;
K = PHT/S;

== matlab function VINS/measUpdate/absolutePoseUpdate/applyErrors/applyXstateErrors/skew ==
  data: inp_vr input; res output
function res=skew(inp_vr)
res=[cast(0, 'like', inp_vr)	-inp_vr(3)                  inp_vr(2); ...
     inp_vr(3)                  cast(0, 'like', inp_vr)     -inp_vr(1);...
	 -inp_vr(2)                 inp_vr(1)                   cast(0, 'like', inp_vr)];

== matlab function VINS/measUpdate/absolutePoseUpdate/calculateKalmanGain ==
  data: chiSquared output; P input; K output; H input; R input; nu input
function [chiSquared,K] = calcKalmanGain(P, H, R, nu)

PHT = P*H';
S = H*PHT + R;
K = PHT/S;

chiSquared = nu' * (S \ nu);

== matlab function VINS/measUpdate/formDelayedInnovation/MATLAB Function3 ==
  data: Cbn input; eul output size=[3,1]
function eul = dcm2euler(Cbn)

%DCM is Cbn (transforms vectors from b to n)
%eul defined as zyx sequence (yaw,pitch,roll),  but listed in
%roll,pitch,yaw order


pitch=asin(-Cbn(3,1));  %pitch is assumed to be [-pi pi]. singular at pi. use ad-hoc methods to remedy this deficiency
roll=atan2(Cbn(3,2), Cbn(3,3));
heading = atan2(Cbn(2,1), Cbn(1,1));
eul=[roll;pitch;heading];

== matlab function VINS/measUpdate/commanded reloc/setYaw1/MATLAB Function3 ==
  data: Cbn input; eul output size=[3,1]
function eul = dcm2euler(Cbn)

%DCM is Cbn (transforms vectors from b to n)
%eul defined as zyx sequence (yaw,pitch,roll),  but listed in
%roll,pitch,yaw order


pitch=asin(-Cbn(3,1));  %pitch is assumed to be [-pi pi]. singular at pi. use ad-hoc methods to remedy this deficiency
roll=atan2(Cbn(3,2), Cbn(3,3));
heading = atan2(Cbn(2,1), Cbn(1,1));
eul=[roll;pitch;heading];

== matlab function VINS/measUpdate/absolutePoseUpdate/updateCovariance/josephCovarianceUpdate ==
  data: P input; Pplus output; K input; H input; R input; IminKH output
function [Pplus, IminKH] = josephCovarianceUpdate(P, K, H, R)

IminKH = eye(size(P), 'like', P) - K*H;
Pplus = IminKH*P*IminKH' + K*R*K';


% re-symmetrize:
Pplus = (Pplus + Pplus')/2;

== matlab function VINS/measUpdate/compass meas update/MATLAB Function3 ==
  data: P input; Pplus output; K input; H input; R input; IminKH output
function [Pplus, IminKH] = josephCovarianceUpdate(P, K, H, R)

IminKH = eye(size(P)) - K*H;
Pplus = IminKH*P*IminKH' + K*R*K';

== matlab function VINS/INS/MATLAB Function ==
  data: DCMbn_old input; DCMbn_new output; w input; Dt input
function DCMbn_new  = bodupdat(DCMbn_old, w, Dt)
%BODUPDAT		Update the direction cosine matrix
%              for body motion (relative to inertial space).
%              The function is thus acting upon the strapdown
%              gyro outputs.
%       
%	DCMbn_new = bodupdat(DCMbn_old,ang_vect)
%     or
%  [DCMbn_new,DCMbb] = bodupdat(DCMbn_old,ang_vect)
%
%   INPUTS
%       DCMbn_old  = current direction cosine matrix providing the
%                    transformation from body to nav coordinates
%
%       ang_vect = incremental integral of body angular
%                  rate vector; in the absence of coning
%                  (i.e., angular rate vector is constant
%                  over the integration interval), this
%                  is the output of the rate-integrating
%                  gyros.
%          ang_vect(1) = x-component (roll);
%          ang_vect(2) = y-component (pitch);
%          ang_vect(3) = z-component (yaw);
%
%   OUTPUTS
%       DCMbn_new = updated direction cosine matrix relating the
%                   current body-frame to the previous
%                   navigation-frame.  Note that the update of
%                   the navigation frame (which is related to
%                   the local-level frame) is accomplished in
%                   function LCLEVUPD
%
%       DCMbb = direction cosine matrix providing the
%               transformation from the body coordinates at
%               time k+1 to the body coordinates at time k
%

%	M. & S. Braasch 4-98
%	Copyright (c) 1997-98 by GPSoft LLC
%	All Rights Reserved.
%

if nargin<3,error('insufficient number of input arguments'),end
ang_vect = w*Dt;

S = skewsymm(ang_vect);
magn = norm(ang_vect);
if magn == 0
   DCMbb = eye(3);
else
   DCMbb = eye(3) + (sin(magn)/magn)*S + ( (1-cos(magn))/magn^2 )*S*S;
end
DCMbn_new = DCMbn_old*DCMbb;

== matlab function VINS/INS/updateDcm ==
  data: Cbn input; Cbn_new output; w input; dt input
function Cbn_new = update_dcm(Cbn, w, dt)

% Update attitude according to TW p.312 approximated to sixth order

rot=w*dt;
rot_norm=norm(rot);
sr_a=1-(rot_norm^2/6)+(rot_norm^4/120);
sr_b=(1/2)-(rot_norm^2/24)+(rot_norm^4/720);
mx_a=eye(3)+sr_a*skew(rot)+sr_b*skew(rot)*skew(rot);

Cbn_new=Cbn*mx_a;


function res=skew(inp_vr)
res=[0 			-inp_vr(3)	inp_vr(2); ...
     inp_vr(3)	0			-inp_vr(1);...
	 -inp_vr(2)	inp_vr(1)	0];

== matlab function VINS/measUpdate/compass meas update/update the Cbn with the errors/MATLAB Function ==
  data: inp_vr input; res output
function res=skew(inp_vr)
res=[0 			-inp_vr(3)	inp_vr(2); ...
     inp_vr(3)	0			-inp_vr(1);...
	 -inp_vr(2)	inp_vr(1)	0];

== matlab function VINS/measUpdate/relativePoseUpdate/formInnovation/MATLAB Function1 ==
  data: Cbn input; eul output size=[3,1]
function eul = dcm2euler(Cbn)

%DCM is Cbn (transforms vectors from b to n)
%eul defined as zyx sequence (yaw,pitch,roll),  but listed in
%roll,pitch,yaw order


pitch=asin(-Cbn(3,1));  %pitch is assumed to be [-pi pi]. singular at pi. use ad-hoc methods to remedy this deficiency
roll=atan2(Cbn(3,2), Cbn(3,3));
heading = atan2(Cbn(2,1), Cbn(1,1));
eul=[roll;pitch;heading];

== matlab function VINS/cameraRelativePosePrediction/localIns/updateDcm ==
  data: Cbn input; Cbn_new output; w input; dt input
function Cbn_new = update_dcm(Cbn, w, dt)

% Update attitude according to TW p.312 approximated to sixth order

rot=w*dt;
rot_norm=norm(rot);
sr_a=1-(rot_norm^2/6)+(rot_norm^4/120);
sr_b=(1/2)-(rot_norm^2/24)+(rot_norm^4/720);
mx_a=eye(3)+sr_a*skew(rot)+sr_b*skew(rot)*skew(rot);

Cbn_new=Cbn*mx_a;


function res=skew(inp_vr)
res=[0 			-inp_vr(3)	inp_vr(2); ...
     inp_vr(3)	0			-inp_vr(1);...
	 -inp_vr(2)	inp_vr(1)	0];

== matlab function VINS/uncomment and set zero noise for verification/plot errors/MATLAB Function1 ==
  data: Cbn input; eul output size=[3,1]
function eul = dcm2euler(Cbn)

%DCM is Cbn (transforms vectors from b to n)
%eul defined as zyx sequence (yaw,pitch,roll),  but listed in
%roll,pitch,yaw order


pitch=asin(-Cbn(3,1));  %pitch is assumed to be [-pi pi]. singular at pi. use ad-hoc methods to remedy this deficiency
roll=atan2(Cbn(3,2), Cbn(3,3));
heading = atan2(Cbn(2,1), Cbn(1,1));
eul=[roll;pitch;heading];

== matlab function VINS/uncomment and set zero noise for verification/plot errors/MATLAB Function2 ==
  data: Cbn input; eul output size=[3,1]
function eul = dcm2euler(Cbn)

%DCM is Cbn (transforms vectors from b to n)
%eul defined as zyx sequence (yaw,pitch,roll),  but listed in
%roll,pitch,yaw order


pitch=asin(-Cbn(3,1));  %pitch is assumed to be [-pi pi]. singular at pi. use ad-hoc methods to remedy this deficiency
roll=atan2(Cbn(3,2), Cbn(3,3));
heading = atan2(Cbn(2,1), Cbn(1,1));
eul=[roll;pitch;heading];

== matlab function VINS/cameraRelativePosePrediction/localIns/MATLAB Function3 ==
  data: Cbn input; eul output size=[3,1]
function eul = dcm2euler(Cbn)

%DCM is Cbn (transforms vectors from b to n)
%eul defined as zyx sequence (yaw,pitch,roll),  but listed in
%roll,pitch,yaw order


pitch=asin(-Cbn(3,1));  %pitch is assumed to be [-pi pi]. singular at pi. use ad-hoc methods to remedy this deficiency
roll=atan2(Cbn(3,2), Cbn(3,3));
heading = atan2(Cbn(2,1), Cbn(1,1));
eul=[roll;pitch;heading];

== matlab function VINS/uncomment and set zero noise for verification/update pure optical pose/MATLAB Function1 ==
  data: Cbn input; eul output size=[3,1]
function eul = dcm2euler(Cbn)

%DCM is Cbn (transforms vectors from b to n)
%eul defined as zyx sequence (yaw,pitch,roll),  but listed in
%roll,pitch,yaw order


pitch=asin(-Cbn(3,1));  %pitch is assumed to be [-pi pi]. singular at pi. use ad-hoc methods to remedy this deficiency
roll=atan2(Cbn(3,2), Cbn(3,3));
heading = atan2(Cbn(2,1), Cbn(1,1));
eul=[roll;pitch;heading];

== matlab function VINS/measUpdate/relativePoseUpdate/updateCovariance/modifiedCholesky ==
  data: G input; L output; D output; E output
%
%  [L,D,E,pneg]=mchol(G)
%
%  Given a symmetric matrix G, find a matrix E of "small" norm and c
%  L, and D such that  G+E is Positive Definite, and 
%
%      G+E = L*D*L'
%
%  Also, calculate a direction pneg, such that if G is not PD, then
%
%      pneg'*G*pneg < 0
%
%  Note that if G is PD, then the routine will return pneg=[]. 
%
%  Reference: Gill, Murray, and Wright, "Practical Optimization", p111.
%  Author: Brian Borchers (borchers@nmt.edu)
%
function [L,D,E]=mchol(G)
%
%  n gives the size of the matrix.
%
n=size(G,1);
%
%  gamma, zi, nu, and beta2 are quantities used by the algorithm.  
%
gamma=max(diag(G));
zi=max(max(G-diag(diag(G))));
nu=max([1,sqrt(n^2-1)]);
beta2=max([gamma, zi/nu, 1.0E-15]);
%
%  Initialize diag(C) to diag(G).
%
C=diag(diag(G));
%
%  Loop through, calculating column j of L for j=1:n
%

L=zeros(n, 'like', G);
D=zeros(n, 'like', G);
E=zeros(n, 'like', G);

for j=1:n
    %
    %  Calculate the jth row of L.  
    %
    if (j > 1)
        L(j,1:j-1)=C(j,1:j-1)./diag(D(1:j-1,1:j-1))';
    end
    %
    %  Update the jth column of C.
    %
    if (j >= 2)
        if (j < n)
            C(j+1:n,j)=G(j+1:n,j)-(L(j,1:j-1)*C(j+1:n,1:j-1)')';
        end
    else
        C(j+1:n,j)=G(j+1:n,j);
    end
    %
    % Update theta. 
    %
    if (j == n)
        theta_j=cast(0, 'like', G);
    else
        theta_j=max(abs(C(j+1:n,j)));
    end
    %
    %  Update D
    %
    D(j,j)=max([eps,abs(C(j,j)),theta_j^2/beta2]');
    %
    % Update E.
    %
    E(j,j)=D(j,j)-C(j,j);

    
    %
    %  Update C again...
    % 
    %%%%%%%% M.Zibulevsky: begin of changes, old version is commented %%%%%%%%%%%%%
    
    %for i=j+1:n,
    %    C(i,i)=C(i,i)-C(i,j)^2/D(j,j);
    %end;
    
    ind=[j*(n+1)+1 : n+1 : n*n]';
    C(ind)=C(ind)-(1/D(j,j))*C(j+1:n,j).^2;


end

%
% Put 1's on the diagonal of L
%
%for j=1:n,
%    L(j,j)=1;
%end;

ind=[1 : n+1 : n*n]';
L(ind)=cast(1, 'like', G);


return

== matlab function VINS/measUpdate/relativePoseUpdate/formMeasurementMatrix/skew1 ==
  data: inp_vr input; res output
function res=skew(inp_vr)
res=[cast(0, 'like', inp_vr)	-inp_vr(3)                  inp_vr(2); ...
     inp_vr(3)                  cast(0, 'like', inp_vr)     -inp_vr(1);...
	 -inp_vr(2)                 inp_vr(1)                   cast(0, 'like', inp_vr)];

== matlab function VINS/cameraRelativePosePrediction/frameToFramePrediction/MATLAB Function3 ==
  data: Cbn input; eul output size=[3,1]
function eul = dcm2euler(Cbn)

%DCM is Cbn (transforms vectors from b to n)
%eul defined as zyx sequence (yaw,pitch,roll),  but listed in
%roll,pitch,yaw order


pitch=asin(-Cbn(3,1));  %pitch is assumed to be [-pi pi]. singular at pi. use ad-hoc methods to remedy this deficiency
roll=atan2(Cbn(3,2), Cbn(3,3));
heading = atan2(Cbn(2,1), Cbn(1,1));
eul=[roll;pitch;heading];

== matlab function VINS/measUpdate/wipe out delayed states/setP/MATLAB Function1 ==
  data: initialRotUncert input; initialPosUncert input; initialVelUncert input; P0 output size=[modelDef.numStates, modelDef.numStates]; modelDef parameter; imuPar parameter; gyroBiasCov input; accelBiasCov input
function P0  = calculate_P0(initialRotUncert, initialPosUncert, initialVelUncert, modelDef, imuPar, gyroBiasCov, accelBiasCov)

% order of the states:
% 1:3   phi
% 4:6   dw
% 7:9   dr
% 10:12 dv
% 13:15 df  (if modelDef.trackAccelBiases)
% 16:24 dM_gyro in column-major order (if modelDef.trackGyroSfma)
% 25:33 dM_accel in column-major order (if modelDef.trackAccelSfma)
% 34:42 dG_gyro in column-major order (if modelDef.trackGyroGsens)

P0 = zeros(modelDef.numStates, 'like', initialRotUncert);

P0(1:3, 1:3) = diag(initialRotUncert.^2);
if any(gyroBiasCov)
    P0(4:6, 4:6) = gyroBiasCov;
else
    P0(4:6, 4:6) = eye(3)*(imuPar.gyroBiasUncert.^2);
end
P0(7:9, 7:9) = diag(initialPosUncert.^2);
P0(10:12, 10:12) = diag(initialVelUncert.^2);


if modelDef.trackAccelBiases
    if any(accelBiasCov)
        P0(13:15, 13:15) = accelBiasCov;
    else
        P0(13:15, 13:15) = eye(3)*(imuPar.accelBiasUncert.^2);
    end
end

if modelDef.trackGyroSfma  
    vec9 = ones(9,1)*imuPar.gyroAlignUncert^2;
    vec9([1 5 9]) = imuPar.gyroScaleUncert^2;
    P0(16:24, 16:24) = diag(vec9);
end

if modelDef.trackAccelSfma  % propagate dM_accel to dv
    vec9 = ones(9,1)*imuPar.accelAlignUncert^2;
    vec9([1 5 9]) = imuPar.accelScaleUncert^2;
    if modelDef.accelDefinesExtrinsics
        vec9([4 7]) = 0.0001^2; % x accel has no misalignment so picks up no component of y or z accelerations
        vec9(8) = 0.0001^2;  % y accel has no tilt out of xy plane, so picks up no component of z acceleration
    end
    P0(25:33, 25:33) = diag(vec9);
end

if modelDef.trackGyroGsens
    vec9 = ones(9,1)*imuPar.gyroGsensUncert^2;
    P0(34:42, 34:42) = diag(vec9);
end
